simulink model "UsartControl2"  (R2016a)
settings: Solver=FixedStepAuto  StartTime=0.0  StopTime=inf  FixedStep=0.001  RelTol=1e-3
undefined symbols (not defined in the file): serial
libraries: instrumentlib x3, simulink x2
settings Model: Creator=LMPC  LastModifiedBy=LMPC

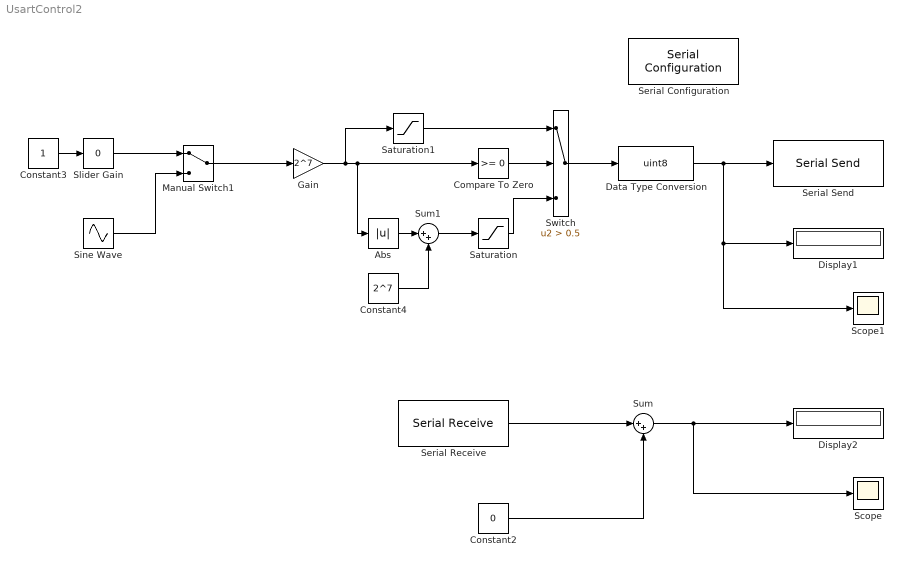
== system UsartControl2 ==
  Abs : Abs
  Compare To Zero : simulink/Logic and Bit Operations/Compare To Zero  relop=>=  OutDataTypeStr=boolean
  Constant2 : Constant  Value=0  OutDataTypeStr=uint8  SampleTime=-1
  Constant3 : Constant  OutDataTypeStr=single  SampleTime=-1
  Constant4 : Constant  Value=2^7  OutDataTypeStr=uint8  SampleTime=-1
  Data Type Conversion : DataTypeConversion  OutDataTypeStr=uint8
  Display1 : Display
      settings: Format=hex (Stored Integer)
  Display2 : Display
      settings: Format=hex (Stored Integer)
  Gain : Gain  Gain=2^7
  Manual Switch1 : ManualSwitch
  Saturation : Saturate  UpperLimit=2^8-1  LowerLimit=0
  Saturation1 : Saturate  UpperLimit=2^7-1  LowerLimit=0
  Scope : Scope
  Scope1 : Scope
  Serial Configuration : instrumentlib/Serial Configuration  Priority=-200000  ComPortMenu=COM1  ComPort=COM1  ObjConstructor=serial('COM1');  BaudRate=57600  DataBits=8  Parity=none  StopBits=1  FlowControl=none  Timeout=10  ByteOrder=LittleEndian
  Serial Receive : instrumentlib/Serial Receive  ComPortMenu=COM1  ComPort=COM1  ObjConstructor=serial('COM1');  Terminator=<none>  DataSize=1  DataType=uint8  EnableBlockingMode=on  ActionDataUnavailable=Output custom value  CustomValue=-25  SampleTime=0.001
  Serial Send : instrumentlib/Serial Send  ComPortMenu=COM1  ComPort=COM1  ObjConstructor=serial('COM1');  Terminator=<none>  EnableBlockingMode=off
  Sine Wave : Sin  SineType=Sample based  Samples=20  SampleTime=0.001
  Slider Gain : simulink/Math Operations/Slider Gain  low=-1  gain=0  high=1
  Sum : Sum  Inputs=|++
  Sum1 : Sum  Inputs=|++
  Switch : Switch  Criteria=u2 > Threshold  Threshold=0.5
  wires:
  Data Type Conversion/1 -> Scope1/1, Display1/1, Serial Send/1
  Sum/1 -> Scope/1, Display2/1
  Constant2/1 -> Sum/2
  Serial Receive/1 -> Sum/1
  Gain/1 -> Compare To Zero/1, Abs/1, Saturation1/1
  Manual Switch1/1 -> Gain/1
  Constant3/1 -> Slider Gain/1
  Switch/1 -> Data Type Conversion/1
  Compare To Zero/1 -> Switch/2
  Abs/1 -> Sum1/1
  Constant4/1 -> Sum1/2
  Sum1/1 -> Saturation/1
  Saturation1/1 -> Switch/1
  Saturation/1 -> Switch/3
  Slider Gain/1 -> Manual Switch1/1
  Sine Wave/1 -> Manual Switch1/2
